simulink model "Adjustedtransfer"  (R2022a)
settings: Solver=VariableStepAuto  StartTime=0.0  StopTime=1e7  RelTol=1e-3
undefined symbols (not defined in the file): denAdjdelay, denAdjZdelay, numAdjdelay, numAdjZdelay, sigbuilder_block
libraries: cstblocks x30, slpidlib x17, slctrlblks x2
(part 2 of 2)

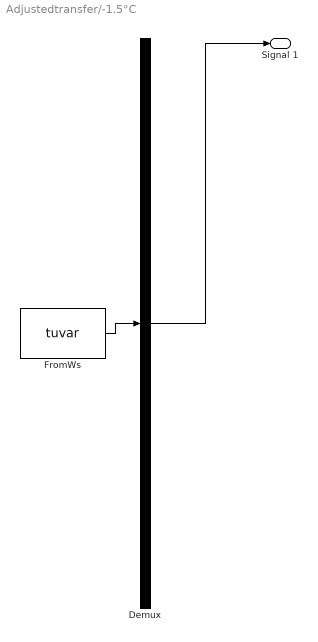
== system Adjustedtransfer/-1.5°C ==
  Demux : Demux  Tag=STV Demux  Outputs=1
      settings: DisplayOption=none
  FromWs : FromWorkspace  Tag=STV FromWs  VariableName=tuvar
      SigBuilderData=|
      | common.afterFinalStr = 'Extrapolate'
      | common.sampleTime = 0
      | dataSet.timeRange = [0 100000]
      | dataSet.name = 'Group 1'
      | sbobj.Groups.Name = 'Group 1'
      | sbobj.Groups.Signals.Name = 'Signal 1'
      | sbobj.Groups.Signals.XData = [0 4 88999 89000 100000]
      | sbobj.Groups.Signals.YData = [-0.5 -0.5 -0.5 -0.0247 -0.0247]
      | sbobj.Groups.TimeRange = [0 100000]
  Signal 1 : Outport  Tag=STV Outport
  wires:
  Demux/1 -> Signal 1/1
  FromWs/1 -> Demux/1

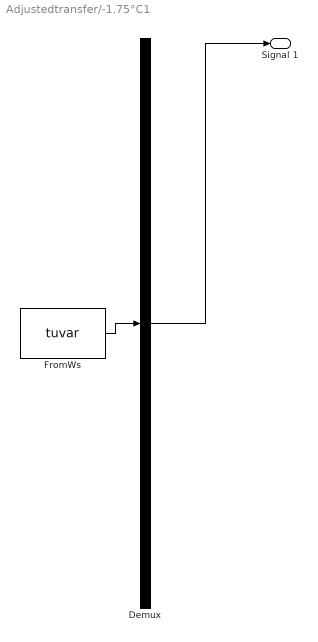
== system Adjustedtransfer/-1.75°C1 ==
  Demux : Demux  Tag=STV Demux  Outputs=1
      settings: DisplayOption=none
  FromWs : FromWorkspace  Tag=STV FromWs  VariableName=tuvar
      SigBuilderData=|
      | common.afterFinalStr = 'Extrapolate'
      | common.sampleTime = 0
      | dataSet.timeRange = [0 100000]
      | dataSet.name = 'Group 1'
      | sbobj.Groups.Name = 'Group 1'
      | sbobj.Groups.Signals.Name = 'Signal 1'
      | sbobj.Groups.Signals.XData = [0 4 88999 89000 100000]
      | sbobj.Groups.Signals.YData = [-0.75 -0.75 -0.75 -0.0247 -0.0247]
      | sbobj.Groups.TimeRange = [0 100000]
  Signal 1 : Outport  Tag=STV Outport
  wires:
  Demux/1 -> Signal 1/1
  FromWs/1 -> Demux/1

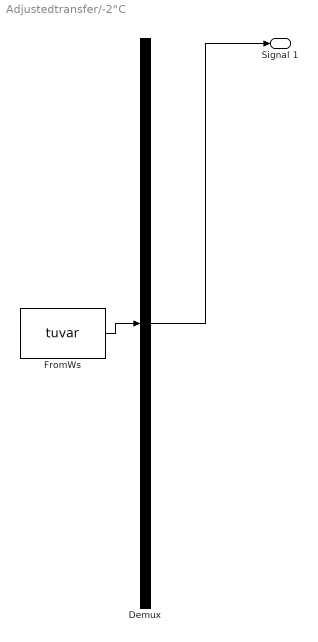
== system Adjustedtransfer/-2°C ==
  Demux : Demux  Tag=STV Demux  Outputs=1
      settings: DisplayOption=none
  FromWs : FromWorkspace  Tag=STV FromWs  VariableName=tuvar
      SigBuilderData=|
      | common.afterFinalStr = 'Extrapolate'
      | common.sampleTime = 0
      | dataSet.timeRange = [0 100000]
      | dataSet.name = 'Group 1'
      | sbobj.Groups.Name = 'Group 1'
      | sbobj.Groups.Signals.Name = 'Signal 1'
      | sbobj.Groups.Signals.XData = [0 4 88999 89000 100000]
      | sbobj.Groups.Signals.YData = [-1 -1 -1 -0.0247 -0.0247]
      | sbobj.Groups.TimeRange = [0 100000]
  Signal 1 : Outport  Tag=STV Outport
  wires:
  Demux/1 -> Signal 1/1
  FromWs/1 -> Demux/1
